simulink model "NPC_new_1"  (R2023a)
settings: Solver=FixedStepAuto  StartTime=0.0  StopTime=0.2  FixedStep=SampleTime  RelTol=1e-3  EnableMultiTasking=on
values from neighbouring files (symbols this model uses):
  Cf = 4e-6    (= 4e-06)    [preload.m]
  L_load = 10e-3    (= 0.01)    [preload.m]
  R_load = 1e-3    (= 0.001)    [preload.m]
  SampleTime = 10e-8    (= 1e-07)    [preload.m]
  Sequence_amplitude = 1    [preload.m]
  Sequence_frequency = fs    (= 2550)    [preload.m]
  V_control_amplitude = ma    (= 0.85)    [preload.m]
  V_control_frequency = V_grid_frequency    (= 314.159265359)    [preload.m]
  V_grid_amplitude = sqrt(2)*240    [preload.m]
  V_grid_frequency = 2*pi*50    (= 314.159265359)    [preload.m]
  Vdc = 752    [preload.m]
undefined symbols (not defined in the file or in its folder): Va_grid_amplitude, Va_grid_frequency, Va_grid_phase
libraries: spsGroundLib x4, spsMosfetLib x4, spsSeriesRLCBranchLib x2, spsDiodeLib x2, spsCurrentMeasurementLib x2, simulink x2, spsVoltageMeasurementLib x2, spsDCVoltageSourceLib x2, spsControlledVoltageSourceLib x1, spspowerguiLib x1
settings Model: Creator=ADMIN  LastModifiedBy=ADMIN
settings DataIOCC: ReturnWorkspaceOutputsName=out_npc

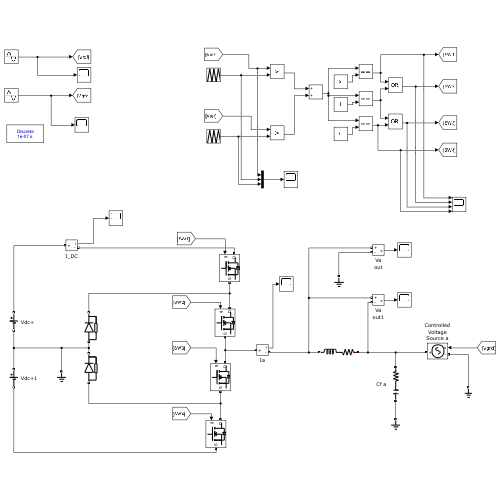
[thumbnail: Simulink's stored preview of the top-level diagram]
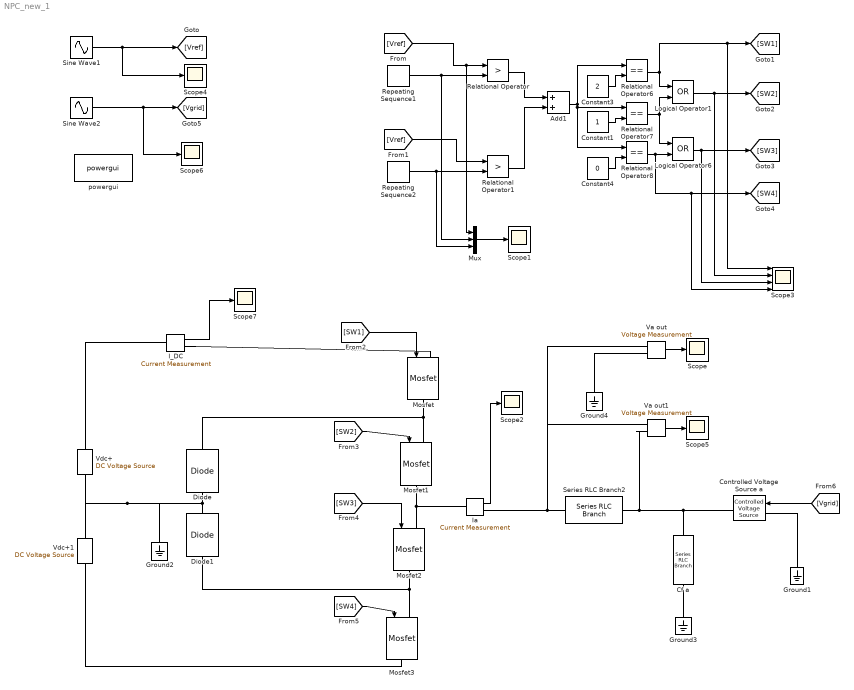
== system NPC_new_1 ==
  Add1 : Sum
  Cf a : spsSeriesRLCBranchLib/Series RLC Branch  LConnTagsString=__new0  RConnTagsString=__new0  BranchType=RC  Resistance=1e-8  Inductance=1e-3  SetiL0=off  InitialCurrent=0  Capacitance=Cf  Setx0=off  InitialVoltage=0  Measurements=None
  Constant1 : Constant
  Constant3 : Constant  Value=2
  Constant4 : Constant  Value=0
  Controlled Voltage Source a : spsControlledVoltageSourceLib/Controlled Voltage Source  Initialize=off  Source_Type=AC  Amplitude=Va_grid_amplitude  Phase=Va_grid_phase  Frequency=Va_grid_frequency  Measurements=None
  Diode : spsDiodeLib/Diode  Ron=0.001  Lon=0  Vf=0.8  IC=0  UseSnubber=0  Rs=500  Cs=250e-9  Measurements=off
  Diode1 : spsDiodeLib/Diode  Ron=0.001  Lon=0  Vf=0.8  IC=0  UseSnubber=0  Rs=500  Cs=250e-9  Measurements=off
  Ground{1..4} (4 alike) : spsGroundLib/Ground  LConnTagsString=a
  I_DC : spsCurrentMeasurementLib/Current Measurement  PhasorSimulation=off  OutputType=Complex  PSBequivalent=0
  Ia : spsCurrentMeasurementLib/Current Measurement  PhasorSimulation=off  OutputType=Complex  PSBequivalent=0
  Logical Operator1 : Logic  Operator=OR  AllPortsSameDT=off  OutDataTypeStr=boolean
  Logical Operator6 : Logic  Operator=OR  AllPortsSameDT=off  OutDataTypeStr=boolean
  Mosfet{,1..3} (4 alike) : spsMosfetLib/Mosfet  Ron=0.1  Lon=0  Rd=0.01  Vfd=0  IC=0  Rs=1e5  Cs=inf  Measurements=off
  Mux : Mux  Inputs=3
  Relational Operator : RelationalOperator  Operator=>  OutDataTypeStr=boolean  RndMeth=Simplest  InputSameDT=off
  Relational Operator1 : RelationalOperator  Operator=>  OutDataTypeStr=boolean  RndMeth=Simplest  InputSameDT=off
  Relational Operator6 : RelationalOperator  Operator===  OutDataTypeStr=boolean  RndMeth=Simplest  InputSameDT=off
  Relational Operator7 : RelationalOperator  Operator===  OutDataTypeStr=boolean  RndMeth=Simplest  InputSameDT=off
  Relational Operator8 : RelationalOperator  Operator===  OutDataTypeStr=boolean  RndMeth=Simplest  InputSameDT=off
  Repeating Sequence1 : simulink/Sources/Repeating Sequence  rep_seq_t=[0 1 2]*[1/Sequence_frequency]  rep_seq_y=[0 Sequence_amplitude 0]
  Repeating Sequence2 : simulink/Sources/Repeating Sequence  rep_seq_t=[0 1 2]*[1/Sequence_frequency]  rep_seq_y=[-Sequence_amplitude 0 -Sequence_amplitude]
  Scope{,1..2,4..7} (7 alike) : Scope
  Scope3 : Scope  NumInputPorts=4
  Series RLC Branch2 : spsSeriesRLCBranchLib/Series RLC Branch  LConnTagsString=__new0  RConnTagsString=__new0  BranchType=RL  Resistance=R_load  Inductance=L_load  SetiL0=off  InitialCurrent=0  Capacitance=1e-6  Setx0=off  InitialVoltage=0  Measurements=None
  Sine Wave1 : Sin  Amplitude=V_control_amplitude  Frequency=V_control_frequency  SampleTime=0
  Sine Wave2 : Sin  Amplitude=V_grid_amplitude  Frequency=V_grid_frequency  SampleTime=0
  Va out : spsVoltageMeasurementLib/Voltage Measurement  PhasorSimulation=off  OutputType=Complex  PSBequivalent=0
  Va out1 : spsVoltageMeasurementLib/Voltage Measurement  PhasorSimulation=off  OutputType=Complex  PSBequivalent=0
  Vdc+ : spsDCVoltageSourceLib/DC Voltage Source  Amplitude=Vdc/2  Measurements=None
  Vdc+1 : spsDCVoltageSourceLib/DC Voltage Source  Amplitude=Vdc/2  Measurements=None
  powergui : spspowerguiLib/powergui  Priority=1  SimulationMode=Discrete  SampleTime=SampleTime  frequency=60  Iterations=50  frequencyindice=0  Pbase=100e6  ErrMax=1e-4  UnitsV=kV  UnitsW=MW  buscounter=0  FunctionMessages=off  echomessages=off  EnableUseOfTLC=off  CurrentSourceSwitches=off  DisableSnubberDevices=off  DisableRonSwitches=off  DisableVfSwitches=off  DisplayEquations=off  AutomaticDiscreteSolvers=off  SolverType=Tustin/Backward Euler (TBE)  Interpol=off  ExternalGateDelay=off  methode=off  Ts=100  x0status=blocks  SPID=on  SwTol=0  HookPort=off  NonlinearTolerance=1e-4  nMaxIteration=100  ContinueOnMaxIteration=off  RestoreLinks=warning  ResistiveCurrentMeasurement=off  Frange=[0:2:500]  Ylog=off  Xlog=on  ShowGrid=off  save=off  variable=ZData  structure=0  ZoomFFT=off  StartTime=0.0  cycles=1  DisplayStyle=1  fundamental=60  FreqAxis=off  MaxFrequency=1000  frequencyindicesteady=1  RmsSteady=1  display=off
  wires:
  Relational Operator7/1 -> Logical Operator6/1, Logical Operator1/2
  Constant1/1 -> Relational Operator7/2
  Constant4/1 -> Relational Operator8/2
  Add1/1 -> Relational Operator8/1, Relational Operator7/1, Relational Operator6/1
  Relational Operator1/1 -> Add1/2
  Constant3/1 -> Relational Operator6/2
  Relational Operator/1 -> Add1/1
  Sine Wave1/1 -> Scope4/1, [Vref]
  Repeating Sequence1/1 -> Mux/2, Relational Operator/2
  Repeating Sequence2/1 -> Mux/3, Relational Operator1/2
  [Vref] -> Relational Operator1/1
  [Vref] -> Mux/1, Relational Operator/1
  [SW1] -> Mosfet/1
  [SW2] -> Mosfet1/1
  [SW3] -> Mosfet2/1
  [SW4] -> Mosfet3/1
  [Vgrid] -> Controlled Voltage Source a/1
  Sine Wave2/1 -> Scope6/1, [Vgrid]
  Relational Operator6/1 -> Logical Operator1/1, [SW1], Scope3/1
  Logical Operator1/1 -> [SW2], Scope3/2
  Logical Operator6/1 -> Scope3/3, [SW3]
  Relational Operator8/1 -> [SW4], Scope3/4, Logical Operator6/2
  Ia/1 -> Scope2/1
  Mux/1 -> Scope1/1
  Va out/1 -> Scope/1
  Va out1/1 -> Scope5/1
  I_DC/1 -> Scope7/1
  connections:
  Vdc+1/LConn1 -- Mosfet3/RConn1
  Mosfet2/RConn1 -- Diode1/LConn1 -- Mosfet3/LConn1
  Mosfet1/RConn1 -- Ia/LConn1 -- Mosfet2/LConn1
  Mosfet/RConn1 -- Mosfet1/LConn1 -- Diode/RConn1
  Ia/RConn1 -- Va out1/LConn1 -- Va out/LConn1 -- Series RLC Branch2/RConn1
  Controlled Voltage Source a/RConn1 -- Cf a/LConn1 -- Va out1/LConn2 -- Series RLC Branch2/LConn1
  Controlled Voltage Source a/LConn1 -- Ground1/LConn1
  Diode/LConn1 -- Ground2/LConn1 -- Vdc+1/RConn1 -- Vdc+/LConn1 -- Diode1/RConn1
  Ground4/LConn1 -- Va out/LConn2
  Ground3/LConn1 -- Cf a/RConn1
  I_DC/RConn1 -- Mosfet/LConn1
  I_DC/LConn1 -- Vdc+/RConn1
